simulink model "gm_sampleModel1519_4_sub"  (R2023a)
settings: Solver=VariableStepAuto  StartTime=0.0  StopTime=10.0  RelTol=1e-3
libraries: simulink x2
settings Model: Creator=user1  LastModifiedBy=user1
settings OptimizationCC: BlockReduction=off  ConditionallyExecuteInputs=off
settings DebuggingCC: InheritedTsInSrcMsg=none

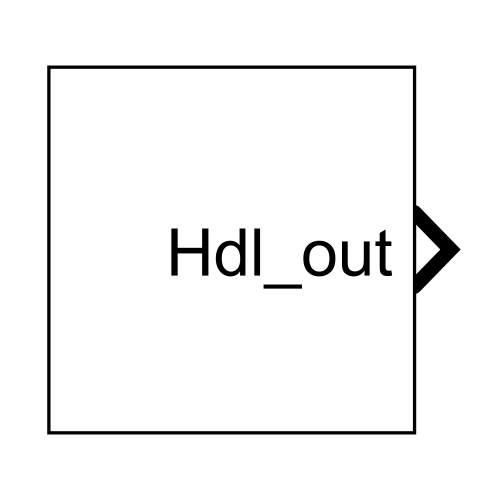
[thumbnail: Simulink's stored preview of the top-level diagram]
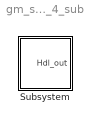
== system gm_sampleModel1519_4_sub ==
  Subsystem : Subsystem

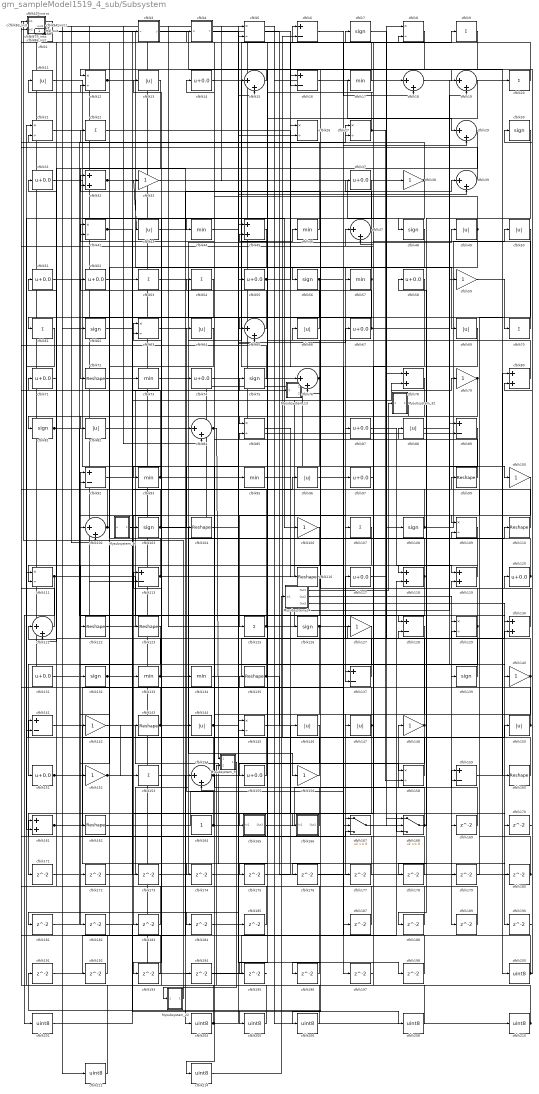
== system gm_sampleModel1519_4_sub/Subsystem ==
  Mysubsystem_13 : Subsystem
  Mysubsystem_22 : Subsystem
  Mysubsystem_32 : Subsystem
  Mysubsystem_34 : Subsystem
  Mysubsystem_36 : Subsystem
  Mysubsystem_9 : Subsystem
  cfblk1 : simulink/Logic and Bit Operations/Detect Increase  vinit=0.0  OutDataTypeStr=uint8
      settings: LibrarySourceBlock=|
      | hdlsllib/Logic and Bit
      | Operations/Detect
      | Increase
  cfblk{33,38,59,79,100,106,127,140,142,148,152,156} (12 alike) : Gain  OutDataTypeStr=uint8
  cfblk{15,18..19,29,39,47,65,76,84,102,121,154} (12 alike) : Sum  Inputs=|++  OutDataTypeStr=uint8
  cfblk{7,30,48,56,62,75,81,103,108,126,132,139} (12 alike) : Signum
  cfblk{72,99,104,110,116,122..123,135,143,160,162} (11 alike) : Reshape
  cfblk105_inst : Subsystem
  cfblk{9,20,22,53..54,61,70,107,125,153} (10 alike) : Sum  Inputs=+  OutDataTypeStr=uint8
  cfblk{5,8,12,21,26..27,42,63,85,109,111,129,145,158} (14 alike) : Product  Inputs=*/  OutDataTypeStr=uint8  RndMeth=Zero  SaturateOnIntegerOverflow=on
  cfblk{11,13,43,49..50,64,66,69,82,88,96,144,146..147,150} (15 alike) : Abs  OutDataTypeStr=uint8  SaturateOnIntegerOverflow=off
  cfblk112_inst : Subsystem
  cfblk{6,16,89,92,113,128,137,141,159} (9 alike) : Sum  Inputs=+-  OutDataTypeStr=uint8
  cfblk114_inst : Subsystem
  cfblk{14,31,37,51..52,55,58,67,71,74,87,97,117,120,131,151,155} (17 alike) : Bias  Bias=0.0  SaturateOnIntegerOverflow=off
  cfblk{32,45,78,80,118..119,130,161} (8 alike) : Sum  OutDataTypeStr=uint8
  cfblk124_inst : Subsystem
  cfblk{17,44,46,57,73,93,95,133..134} (9 alike) : MinMax  OutDataTypeStr=uint8
  cfblk149_inst : Subsystem
  cfblk157_inst : Subsystem
  cfblk164 : Constant  OutDataTypeStr=uint8  SampleTime=-1
  cfblk165 : Subsystem
  cfblk166 : Subsystem
  cfblk167 : Switch  OutDataTypeStr=uint8  SaturateOnIntegerOverflow=off  InputSameDT=off
  cfblk168 : Switch  OutDataTypeStr=uint8  SaturateOnIntegerOverflow=off  InputSameDT=off
  cfblk{169..185,187..198} (29 alike) : Delay  SampleTime=1
  cfblk{200..201,204..206,208,210,212,214} (9 alike) : DataTypeConversion  OutDataTypeStr=uint8  SaturateOnIntegerOverflow=off  RndMeth=Floor
  cfblk24_inst : Subsystem
  cfblk25_inst : Subsystem
  cfblk3 : Subsystem  mask(Compare To Zero){relop=<=, OutDataTypeStr=uint8, ZeroCross=on}
      mask prompts: relop "Simulink:masks:Operator_MP"; OutDataTypeStr "Simulink:masks:OutputDataType_MP"; ZeroCross "Simulink:masks:EnableZerocrossingDetection_MP"
      mask help: Simulink:masks:CompareToZero_MD
      mask init:
      | OutDataTypeStr = 'uint8';
      | ZeroCross = 'on';
      | blkName = 'sampleModel1519_4_sub/Subsystem/cfblk3';
      | relop = '<=';
      | setValue = 'fixdt(0, 8)';
      mask TypeOptions relop: == | ~= | < | <= | >= | >
      mask TypeOptions OutDataTypeStr: Simulink:masks:uint8 | Simulink:masks:boolean
      mask Callback ZeroCross: sl('zeroCrossEnable', gcbh);
      mask Display: disp([relop,' 0'])
  cfblk34_inst : Subsystem
  cfblk36_inst : Subsystem
  cfblk4 : Subsystem  mask(Detect Rise Positive){vinit=double(0), InputProcessing=Elements as channels (sample based), OutDataTypeStr=uint8}
      mask prompts: vinit "Simulink:masks:InitialCondition_MP"; InputProcessing "Simulink:masks:InputProcessing_MP"; OutDataTypeStr "Simulink:masks:OutputDataType_MP"
      mask help: Simulink:masks:DetectRisePositive_MD
      mask init:
      | InputProcessing = 'Elements as channels (sample based)';
      | OutDataTypeStr = 'uint8';
      | vinit = double(0);
      mask TypeOptions InputProcessing: Simulink:masks:ColumnsAsChannelsFrameBased | Simulink:masks:ElementsAsChannelsSampleBased
      mask TypeOptions OutDataTypeStr: Simulink:masks:uint8 | Simulink:masks:boolean
      mask Display: fprintf('U > 0\n&  NOT\nU/z > 0')
  cfblk41_inst : Subsystem
  cfblk77_inst : Subsystem
  cfblk83_inst : Subsystem
  cfblk86_inst : Subsystem
  cfblk94_inst : Subsystem
  Hdl_out : Outport  OutDataTypeStr=uint8  SampleTime=1
  wires:
  Mysubsystem_13/1(Out1) -> Mysubsystem_36/1(u)
  Mysubsystem_13/2(Out2) -> cfblk184/1
  Mysubsystem_22/1(Out1) -> cfblk34_inst/1(in1)
  Mysubsystem_32/1(Out1) -> cfblk191/1
  Mysubsystem_34/1(Out1) -> Mysubsystem_32/1(In1)
  Mysubsystem_34/2(Out2) -> cfblk189/1
  Mysubsystem_34/3(Out3) -> cfblk190/1
  Mysubsystem_36/1(Out1) -> cfblk183/1
  Mysubsystem_9/1(Out1) -> Mysubsystem_22/1(In1)
  cfblk1/1 -> cfblk44/1
  cfblk100/1 -> cfblk125/1
  cfblk102/1 -> cfblk25_inst/2(in2), cfblk27/1
  cfblk103/1 -> cfblk114_inst/2(in2), cfblk156/1, cfblk109/2
  cfblk104/1 -> cfblk145/1
  cfblk105_inst/1(out1) -> cfblk149_inst/2(in2)
  cfblk106/1 -> cfblk111/2
  cfblk107/1 -> cfblk165/1(In1)
  cfblk108/1 -> cfblk92/1, cfblk50/1
  cfblk109/1 -> cfblk182/1
  cfblk11/1 -> cfblk185/1
  cfblk110/1 -> cfblk24_inst/2(in2)
  cfblk111/1 -> cfblk201/1, cfblk130/1
  cfblk112_inst/1(out1) -> cfblk84/2, cfblk212/1
  cfblk113/1 -> cfblk78/2, cfblk11/1
  cfblk114_inst/1(out1) -> cfblk53/1
  cfblk116/1 -> cfblk172/1
  cfblk117/1 -> cfblk8/1
  cfblk118/1 -> cfblk71/1, cfblk12/2, cfblk153/1
  cfblk119/1 -> cfblk118/1
  cfblk12/1 -> cfblk69/1, cfblk137/2
  cfblk120/1 -> cfblk94_inst/1(in1), cfblk157_inst/2(in2)
  cfblk121/1 -> cfblk83_inst/2(in2)
  cfblk122/1 -> cfblk75/1
  cfblk123/1 -> cfblk132/1
  cfblk124_inst/1(out1) -> cfblk38/1
  cfblk125/1 -> cfblk19/2, cfblk13/1
  cfblk126/1 -> cfblk214/1, cfblk130/2
  cfblk127/1 -> cfblk151/1
  cfblk128/1 -> cfblk177/1
  cfblk129/1 -> cfblk88/1, cfblk76/2, cfblk155/1
  cfblk13/1 -> cfblk72/1
  cfblk130/1 -> cfblk32/1
  cfblk131/1 -> cfblk133/1
  cfblk132/1 -> cfblk79/1, cfblk179/1
  cfblk133/1 -> cfblk92/2, cfblk49/1
  cfblk134/1 -> cfblk78/1
  cfblk135/1 -> cfblk64/1, cfblk146/1
  cfblk137/1 -> cfblk157_inst/1(in1)
  cfblk139/1 -> cfblk58/1
  cfblk14/1 -> cfblk168/1
  cfblk140/1 -> cfblk99/1, cfblk154/2
  cfblk141/1 -> cfblk194/1
  cfblk142/1 -> cfblk180/1
  cfblk143/1 -> cfblk6/1, cfblk21/2
  cfblk144/1 -> cfblk67/1, cfblk14/1
  cfblk145/1 -> cfblk169/1
  cfblk146/1 -> cfblk181/1
  cfblk147/1 -> cfblk7/1, cfblk51/1, cfblk85/2, cfblk171/1
  cfblk148/1 -> cfblk117/1, cfblk176/1
  cfblk149_inst/1(out1) -> cfblk131/1
  cfblk15/1 -> cfblk12/1
  cfblk150/1 -> cfblk41_inst/2(in2), cfblk27/2
  cfblk151/1 -> cfblk150/1, cfblk73/1
  cfblk152/1 -> cfblk96/1, cfblk143/1
  cfblk153/1 -> cfblk46/1
  cfblk154/1 -> cfblk113/1, cfblk26/2
  cfblk155/1 -> cfblk21/1
  cfblk156/1 -> cfblk74/1
  cfblk157_inst/1(out1) -> cfblk126/1
  cfblk158/1 -> cfblk135/1
  cfblk159/1 -> cfblk80/1
  cfblk16/1 -> cfblk29/1
  cfblk160/1 -> cfblk141/1
  cfblk161/1 -> cfblk15/2, cfblk17/1
  cfblk162/1 -> cfblk97/1
  cfblk164/1 -> cfblk144/1, cfblk110/1
  cfblk165/1(Out1) -> cfblk148/1
  cfblk166/1(Out1) -> cfblk86_inst/1(in1)
  cfblk167/1 -> cfblk159/1
  cfblk168/1 -> cfblk128/2, cfblk42/1, cfblk127/1
  cfblk169/1 -> cfblk159/2
  cfblk17/1 -> cfblk36_inst/2(in2)
  cfblk170/1 -> cfblk19/1
  cfblk171/1 -> cfblk167/3
  cfblk172/1 -> cfblk65/2
  cfblk173/1 -> cfblk6/2
  cfblk174/1 -> cfblk5/2
  cfblk175/1 -> cfblk18/1
  cfblk176/1 -> cfblk29/2
  cfblk177/1 -> cfblk105_inst/1(in1)
  cfblk178/1 -> cfblk45/2
  cfblk179/1 -> cfblk119/2
  cfblk18/1 -> cfblk140/1
  cfblk180/1 -> cfblk129/2, Hdl_out/1
  cfblk181/1 -> cfblk26/1
  cfblk182/1 -> cfblk205/1
  cfblk183/1 -> cfblk77_inst/2(in2)
  cfblk184/1 -> cfblk39/2
  cfblk185/1 -> cfblk161/1
  cfblk187/1 -> cfblk36_inst/1(in1)
  cfblk188/1 -> cfblk121/1
  cfblk189/1 -> cfblk112_inst/2(in2)
  cfblk19/1 -> cfblk65/1
  cfblk190/1 -> cfblk80/2
  cfblk191/1 -> cfblk154/1
  cfblk192/1 -> cfblk124_inst/2(in2)
  cfblk193/1 -> cfblk83_inst/1(in1)
  cfblk194/1 -> cfblk118/2
  cfblk195/1 -> cfblk1/1
  cfblk196/1 -> cfblk149_inst/1(in1)
  cfblk197/1 -> cfblk47/2
  cfblk198/1 -> cfblk167/2
  cfblk20/1 -> cfblk124_inst/1(in1)
  cfblk200/1 -> cfblk30/1, cfblk120/1, cfblk102/1
  cfblk201/1 -> cfblk3/1(u)
  cfblk204/1 -> cfblk77_inst/1(in1), cfblk15/1
  cfblk205/1 -> cfblk63/1
  cfblk206/1 -> cfblk63/2
  cfblk208/1 -> Mysubsystem_9/2(In2)
  cfblk21/1 -> cfblk84/1
  cfblk210/1 -> cfblk86_inst/2(in2), cfblk47/1, cfblk111/1
  cfblk212/1 -> cfblk34_inst/2(in2)
  cfblk214/1 -> Mysubsystem_34/1(In1)
  cfblk22/1 -> cfblk87/1
  cfblk24_inst/1(out1) -> cfblk162/1
  cfblk25_inst/1(out1) -> cfblk62/1, cfblk113/2
  cfblk26/1 -> cfblk56/1
  cfblk27/1 -> cfblk25_inst/1(in1), cfblk158/2
  cfblk29/1 -> cfblk121/2
  cfblk3/1(y) -> cfblk200/1
  cfblk30/1 -> cfblk188/1
  cfblk31/1 -> cfblk106/1
  cfblk32/1 -> cfblk43/1, cfblk95/1
  cfblk33/1 -> cfblk108/1
  cfblk34_inst/1(out1) -> cfblk210/1
  cfblk36_inst/1(out1) -> cfblk76/1, cfblk102/2
  cfblk37/1 -> cfblk103/1
  cfblk38/1 -> cfblk48/1, cfblk141/2, cfblk22/1
  cfblk39/1 -> cfblk24_inst/1(in1)
  cfblk4/1(Y) -> cfblk158/1
  cfblk41_inst/1(out1) -> cfblk123/1
  cfblk42/1 -> cfblk174/1, cfblk173/1
  cfblk43/1 -> cfblk39/1
  cfblk44/1 -> cfblk139/1
  cfblk45/1 -> cfblk152/1
  cfblk46/1 -> cfblk105_inst/2(in2)
  cfblk47/1 -> cfblk37/1, cfblk57/1
  cfblk48/1 -> cfblk85/1
  cfblk49/1 -> cfblk206/1, cfblk4/1(U)
  cfblk5/1 -> cfblk16/2
  cfblk50/1 -> cfblk109/1
  cfblk51/1 -> cfblk89/1
  cfblk52/1 -> cfblk129/1
  cfblk53/1 -> cfblk160/1
  cfblk54/1 -> cfblk82/1
  cfblk55/1 -> cfblk197/1, cfblk195/1, cfblk9/1
  cfblk56/1 -> cfblk8/2, cfblk61/1, cfblk93/1
  cfblk57/1 -> cfblk114_inst/1(in1), cfblk193/1
  cfblk58/1 -> cfblk167/1
  cfblk59/1 -> cfblk70/1
  cfblk6/1 -> cfblk18/2
  cfblk61/1 -> cfblk161/2
  cfblk62/1 -> cfblk33/1
  cfblk63/1 -> cfblk204/1
  cfblk64/1 -> cfblk142/1
  cfblk65/1 -> cfblk45/1
  cfblk66/1 -> cfblk52/1
  cfblk67/1 -> cfblk59/1, cfblk42/2
  cfblk69/1 -> cfblk137/1
  cfblk7/1 -> cfblk168/2
  cfblk70/1 -> cfblk16/1
  cfblk71/1 -> cfblk31/1
  cfblk72/1 -> cfblk166/1(In1)
  cfblk73/1 -> cfblk208/1
  cfblk74/1 -> cfblk55/1
  cfblk75/1 -> cfblk41_inst/1(in1)
  cfblk76/1 -> cfblk104/1, cfblk5/1
  cfblk77_inst/1(out1) -> cfblk112_inst/1(in1)
  cfblk78/1 -> cfblk122/1
  cfblk79/1 -> cfblk81/1, cfblk178/1
  cfblk8/1 -> cfblk175/1
  cfblk80/1 -> cfblk66/1
  cfblk81/1 -> cfblk128/1, cfblk107/1
  cfblk82/1 -> cfblk134/1
  cfblk83_inst/1(out1) -> cfblk20/1
  cfblk84/1 -> Mysubsystem_9/1(In1), cfblk54/1
  cfblk85/1 -> cfblk116/1
  cfblk86_inst/1(out1) -> cfblk89/2
  cfblk87/1 -> cfblk119/1
  cfblk88/1 -> cfblk100/1
  cfblk89/1 -> cfblk145/2
  cfblk9/1 -> cfblk196/1
  cfblk92/1 -> Mysubsystem_13/1(In1)
  cfblk93/1 -> cfblk94_inst/2(in2), cfblk168/3, cfblk198/1
  cfblk94_inst/1(out1) -> cfblk192/1
  cfblk95/1 -> cfblk187/1
  cfblk96/1 -> cfblk170/1
  cfblk97/1 -> cfblk147/1
  cfblk99/1 -> cfblk32/2

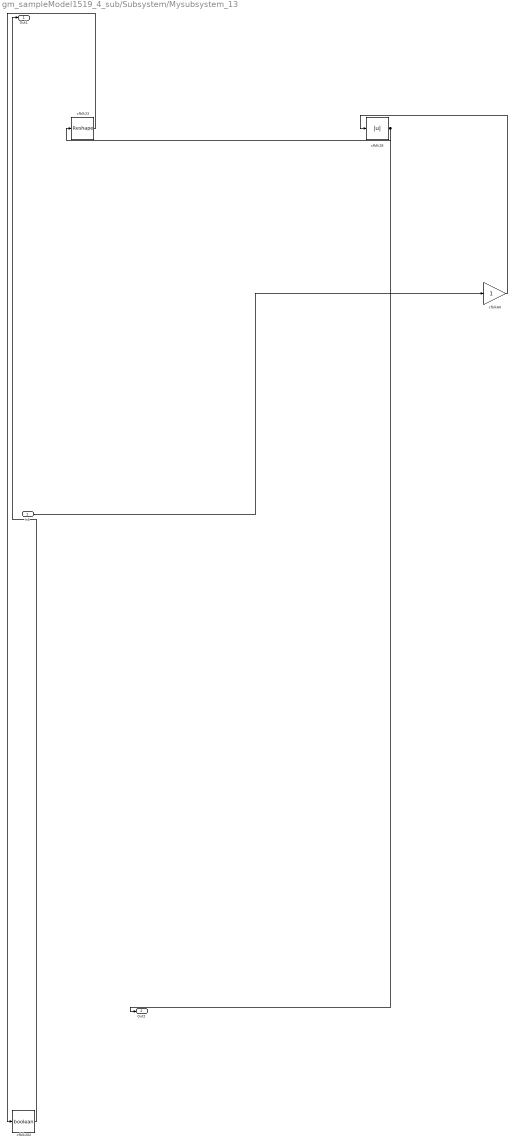
== system gm_sampleModel1519_4_sub/Subsystem/Mysubsystem_13 ==
  In1 : Inport  OutDataTypeStr=uint8  PortDimensions=1  SampleTime=1
  cfblk202 : DataTypeConversion  OutDataTypeStr=boolean  SaturateOnIntegerOverflow=off  RndMeth=Floor
  cfblk23 : Reshape
  cfblk28 : Abs  SaturateOnIntegerOverflow=off
  cfblk60 : Gain
  Out1 : Outport  SampleTime=1
  Out2 : Outport  Port=2  SampleTime=1
  wires:
  In1/1 -> cfblk60/1
  cfblk202/1 -> Out1/1
  cfblk23/1 -> cfblk202/1
  cfblk28/1 -> cfblk23/1, Out2/1
  cfblk60/1 -> cfblk28/1

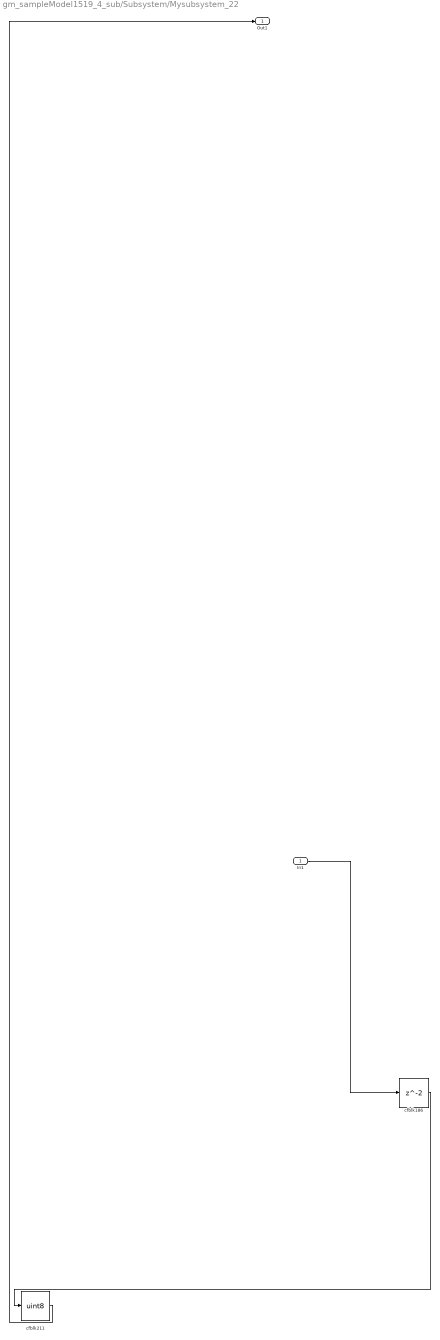
== system gm_sampleModel1519_4_sub/Subsystem/Mysubsystem_22 ==
  In1 : Inport  OutDataTypeStr=uint8  PortDimensions=1  SampleTime=1
  cfblk186 : Delay  SampleTime=1
  cfblk211 : DataTypeConversion  OutDataTypeStr=uint8  SaturateOnIntegerOverflow=off  RndMeth=Floor
  Out1 : Outport  SampleTime=1
  wires:
  In1/1 -> cfblk186/1
  cfblk186/1 -> cfblk211/1
  cfblk211/1 -> Out1/1

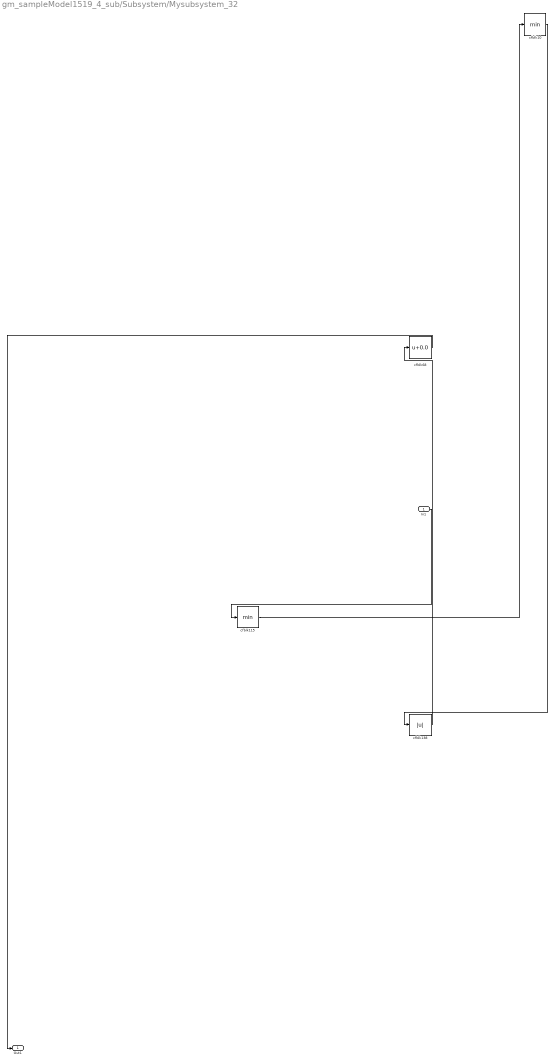
== system gm_sampleModel1519_4_sub/Subsystem/Mysubsystem_32 ==
  In1 : Inport  OutDataTypeStr=uint8  PortDimensions=1  SampleTime=1
  cfblk10 : MinMax
  cfblk115 : MinMax
  cfblk138 : Abs  SaturateOnIntegerOverflow=off
  cfblk68 : Bias  Bias=0.0  SaturateOnIntegerOverflow=off
  Out1 : Outport  SampleTime=1
  wires:
  In1/1 -> cfblk115/1
  cfblk10/1 -> cfblk138/1
  cfblk115/1 -> cfblk10/1
  cfblk138/1 -> cfblk68/1
  cfblk68/1 -> Out1/1

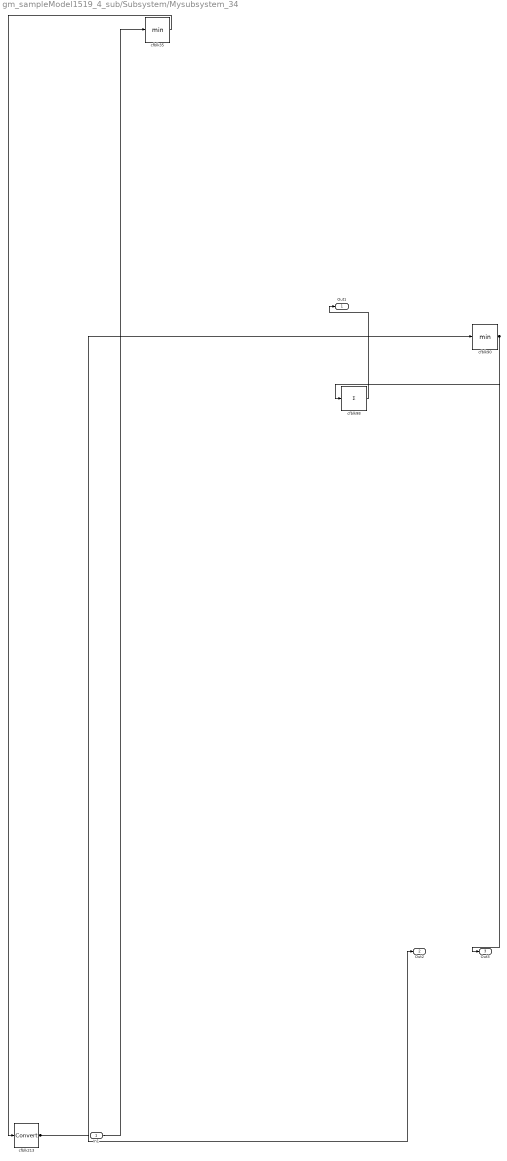
== system gm_sampleModel1519_4_sub/Subsystem/Mysubsystem_34 ==
  In1 : Inport  OutDataTypeStr=uint8  PortDimensions=1  SampleTime=1
  cfblk213 : DataTypeConversion  SaturateOnIntegerOverflow=off  RndMeth=Floor
  cfblk35 : MinMax
  cfblk90 : MinMax
  cfblk98 : Sum  Inputs=+
  Out1 : Outport  SampleTime=1
  Out2 : Outport  Port=2  SampleTime=1
  Out3 : Outport  Port=3  SampleTime=1
  wires:
  In1/1 -> cfblk35/1
  cfblk213/1 -> Out2/1, cfblk90/1
  cfblk35/1 -> cfblk213/1
  cfblk90/1 -> Out3/1, cfblk98/1
  cfblk98/1 -> Out1/1

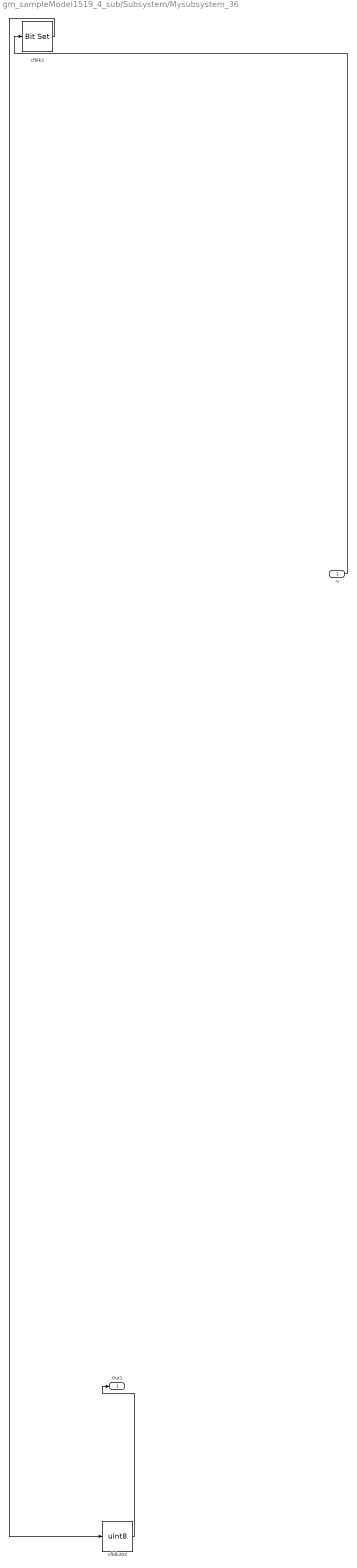
== system gm_sampleModel1519_4_sub/Subsystem/Mysubsystem_36 ==
  u : Inport  OutDataTypeStr=boolean  PortDimensions=1  SampleTime=1
  cfblk2 : simulink/Logic and Bit Operations/Bit Set  iBit=0
      settings: LibrarySourceBlock=|
      | hdlsllib/Logic and Bit
      | Operations/Bit Set
  cfblk203 : DataTypeConversion  OutDataTypeStr=uint8  SaturateOnIntegerOverflow=off  RndMeth=Floor
  Out1 : Outport  SampleTime=1
  wires:
  u/1 -> cfblk2/1
  cfblk2/1 -> cfblk203/1
  cfblk203/1 -> Out1/1

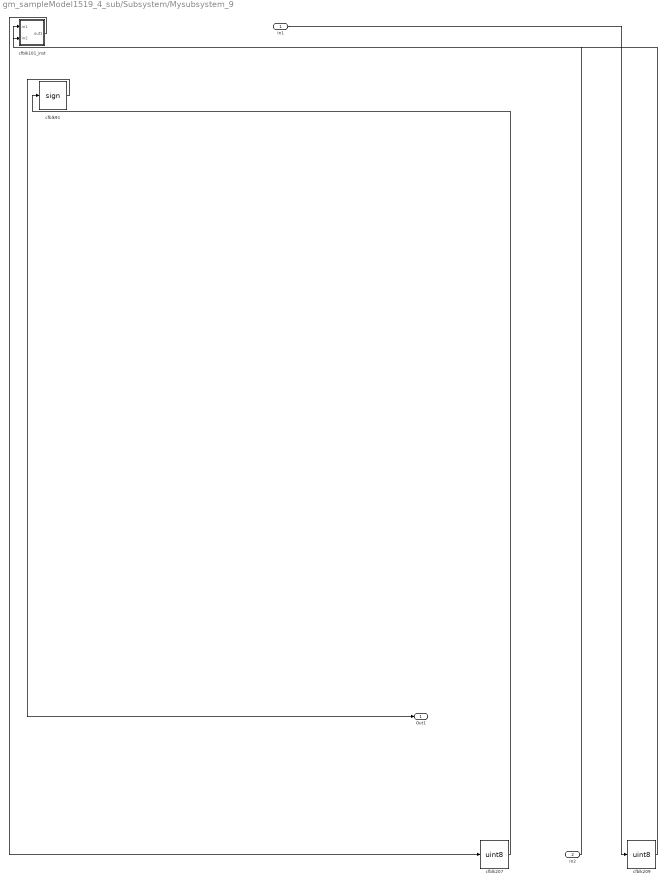
== system gm_sampleModel1519_4_sub/Subsystem/Mysubsystem_9 ==
  In1 : Inport  OutDataTypeStr=uint8  PortDimensions=1  SampleTime=1
  In2 : Inport  Port=2  OutDataTypeStr=uint8  PortDimensions=1  SampleTime=1
  cfblk101_inst : Subsystem
  cfblk207 : DataTypeConversion  OutDataTypeStr=uint8  SaturateOnIntegerOverflow=off  RndMeth=Floor
  cfblk209 : DataTypeConversion  OutDataTypeStr=uint8  SaturateOnIntegerOverflow=off  RndMeth=Floor
  cfblk91 : Signum
  Out1 : Outport  SampleTime=1
  wires:
  In1/1 -> cfblk209/1
  In2/1 -> cfblk101_inst/1(in1)
  cfblk101_inst/1(out1) -> cfblk207/1
  cfblk207/1 -> cfblk91/1
  cfblk209/1 -> cfblk101_inst/2(in2)
  cfblk91/1 -> Out1/1

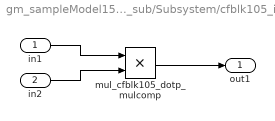
== system gm_sampleModel1519_4_sub/Subsystem/cfblk105_inst ==
  in1 : Inport  OutDataTypeStr=uint8  SampleTime=1
  in2 : Inport  Port=2  OutDataTypeStr=uint8  SampleTime=1
  mul_cfblk105_dotp_mulcomp : Product  Inputs=**  OutDataTypeStr=uint8  SampleTime=1
  out1 : Outport  OutDataTypeStr=uint8  SampleTime=1
  wires:
  in1/1 -> mul_cfblk105_dotp_mulcomp/1
  in2/1 -> mul_cfblk105_dotp_mulcomp/2
  mul_cfblk105_dotp_mulcomp/1 -> out1/1

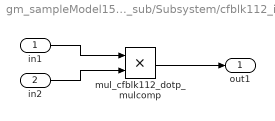
== system gm_sampleModel1519_4_sub/Subsystem/cfblk112_inst ==
  in1 : Inport  OutDataTypeStr=uint8  SampleTime=1
  in2 : Inport  Port=2  OutDataTypeStr=uint8  SampleTime=1
  mul_cfblk112_dotp_mulcomp : Product  Inputs=**  OutDataTypeStr=uint8  SampleTime=1
  out1 : Outport  OutDataTypeStr=uint8  SampleTime=1
  wires:
  in1/1 -> mul_cfblk112_dotp_mulcomp/1
  in2/1 -> mul_cfblk112_dotp_mulcomp/2
  mul_cfblk112_dotp_mulcomp/1 -> out1/1

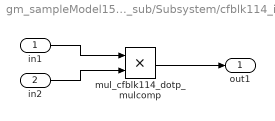
== system gm_sampleModel1519_4_sub/Subsystem/cfblk114_inst ==
  in1 : Inport  OutDataTypeStr=uint8  SampleTime=1
  in2 : Inport  Port=2  OutDataTypeStr=uint8  SampleTime=1
  mul_cfblk114_dotp_mulcomp : Product  Inputs=**  OutDataTypeStr=uint8  SampleTime=1
  out1 : Outport  OutDataTypeStr=uint8  SampleTime=1
  wires:
  in1/1 -> mul_cfblk114_dotp_mulcomp/1
  in2/1 -> mul_cfblk114_dotp_mulcomp/2
  mul_cfblk114_dotp_mulcomp/1 -> out1/1

== system gm_sampleModel1519_4_sub/Subsystem/cfblk124_inst ==
  in1 : Inport  OutDataTypeStr=uint8  SampleTime=1
  in2 : Inport  Port=2  OutDataTypeStr=uint8  SampleTime=1
  mul_cfblk124_dotp_mulcomp : Product  Inputs=**  OutDataTypeStr=uint8  SampleTime=1
  out1 : Outport  OutDataTypeStr=uint8  SampleTime=1
  wires:
  in1/1 -> mul_cfblk124_dotp_mulcomp/1
  in2/1 -> mul_cfblk124_dotp_mulcomp/2
  mul_cfblk124_dotp_mulcomp/1 -> out1/1

== system gm_sampleModel1519_4_sub/Subsystem/cfblk149_inst ==
  in1 : Inport  OutDataTypeStr=uint8  SampleTime=1
  in2 : Inport  Port=2  OutDataTypeStr=uint8  SampleTime=1
  mul_cfblk149_dotp_mulcomp : Product  Inputs=**  OutDataTypeStr=uint8  SampleTime=1
  out1 : Outport  OutDataTypeStr=uint8  SampleTime=1
  wires:
  in1/1 -> mul_cfblk149_dotp_mulcomp/1
  in2/1 -> mul_cfblk149_dotp_mulcomp/2
  mul_cfblk149_dotp_mulcomp/1 -> out1/1

== system gm_sampleModel1519_4_sub/Subsystem/cfblk157_inst ==
  in1 : Inport  OutDataTypeStr=uint8  SampleTime=1
  in2 : Inport  Port=2  OutDataTypeStr=uint8  SampleTime=1
  mul_cfblk157_dotp_mulcomp : Product  Inputs=**  OutDataTypeStr=uint8  SampleTime=1
  out1 : Outport  OutDataTypeStr=uint8  SampleTime=1
  wires:
  in1/1 -> mul_cfblk157_dotp_mulcomp/1
  in2/1 -> mul_cfblk157_dotp_mulcomp/2
  mul_cfblk157_dotp_mulcomp/1 -> out1/1

== system gm_sampleModel1519_4_sub/Subsystem/cfblk165 ==
  In1 : Inport  OutDataTypeStr=uint8  PortDimensions=1  SampleTime=1
  Out1 : Outport  SampleTime=1
  wires:
  In1/1 -> Out1/1

== system gm_sampleModel1519_4_sub/Subsystem/cfblk166 ==
  In1 : Inport  OutDataTypeStr=uint8  PortDimensions=1  SampleTime=1
  Out1 : Outport  SampleTime=1
  wires:
  In1/1 -> Out1/1

== system gm_sampleModel1519_4_sub/Subsystem/cfblk24_inst ==
  in1 : Inport  OutDataTypeStr=uint8  SampleTime=1
  in2 : Inport  Port=2  OutDataTypeStr=uint8  SampleTime=1
  mul_cfblk24_dotp_mulcomp : Product  Inputs=**  OutDataTypeStr=uint8  SampleTime=1
  out1 : Outport  OutDataTypeStr=uint8  SampleTime=1
  wires:
  in1/1 -> mul_cfblk24_dotp_mulcomp/1
  in2/1 -> mul_cfblk24_dotp_mulcomp/2
  mul_cfblk24_dotp_mulcomp/1 -> out1/1

== system gm_sampleModel1519_4_sub/Subsystem/cfblk25_inst ==
  in1 : Inport  OutDataTypeStr=uint8  SampleTime=1
  in2 : Inport  Port=2  OutDataTypeStr=uint8  SampleTime=1
  mul_cfblk25_dotp_mulcomp : Product  Inputs=**  OutDataTypeStr=uint8  SampleTime=1
  out1 : Outport  OutDataTypeStr=uint8  SampleTime=1
  wires:
  in1/1 -> mul_cfblk25_dotp_mulcomp/1
  in2/1 -> mul_cfblk25_dotp_mulcomp/2
  mul_cfblk25_dotp_mulcomp/1 -> out1/1

== system gm_sampleModel1519_4_sub/Subsystem/cfblk3 ==
  u : Inport  OutDataTypeStr=uint8  SampleTime=1
  Compare : RelationalOperator  Operator=<=  OutDataTypeStr=fixdt(0, 8)
  Constant : Constant  DisableCoverage=on  Value=0  OutDataTypeStr=Inherit: Inherit via back propagation  SampleTime=-1  PreserveConstantTs=on
  y : Outport  SampleTime=1
  wires:
  u/1 -> Compare/1
  Compare/1 -> y/1
  Constant/1 -> Compare/2

== system gm_sampleModel1519_4_sub/Subsystem/cfblk34_inst ==
  in1 : Inport  OutDataTypeStr=uint8  SampleTime=1
  in2 : Inport  Port=2  OutDataTypeStr=uint8  SampleTime=1
  mul_cfblk34_dotp_mulcomp : Product  Inputs=**  OutDataTypeStr=uint8  SampleTime=1
  out1 : Outport  OutDataTypeStr=uint8  SampleTime=1
  wires:
  in1/1 -> mul_cfblk34_dotp_mulcomp/1
  in2/1 -> mul_cfblk34_dotp_mulcomp/2
  mul_cfblk34_dotp_mulcomp/1 -> out1/1

== system gm_sampleModel1519_4_sub/Subsystem/cfblk36_inst ==
  in1 : Inport  OutDataTypeStr=uint8  SampleTime=1
  in2 : Inport  Port=2  OutDataTypeStr=uint8  SampleTime=1
  mul_cfblk36_dotp_mulcomp : Product  Inputs=**  OutDataTypeStr=uint8  SampleTime=1
  out1 : Outport  OutDataTypeStr=uint8  SampleTime=1
  wires:
  in1/1 -> mul_cfblk36_dotp_mulcomp/1
  in2/1 -> mul_cfblk36_dotp_mulcomp/2
  mul_cfblk36_dotp_mulcomp/1 -> out1/1

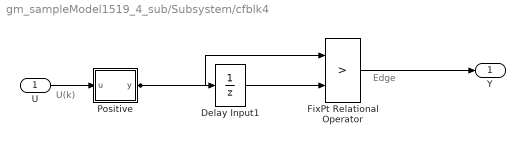
== system gm_sampleModel1519_4_sub/Subsystem/cfblk4 ==
  note: U(k)
  note: Edge
  U : Inport  OutDataTypeStr=uint8  SampleTime=1
  Delay Input1 : UnitDelay  Description=Store in Global RAM  DisableCoverage=on  InitialCondition=vinit  SampleTime=-1  HasFrameUpgradeWarning=on
  FixPt Relational Operator : RelationalOperator  Operator=>  OutDataTypeStr=fixdt(0, 8)  ZeroCross=off  InputSameDT=off
  Positive : Subsystem  mask(Compare To Zero){relop=>, OutDataTypeStr=boolean, ZeroCross=off}
      mask prompts: relop "Simulink:masks:Operator_MP"; OutDataTypeStr "Simulink:masks:OutputDataType_MP"; ZeroCross "Simulink:masks:EnableZerocrossingDetection_MP"
      mask help: Simulink:masks:CompareToZero_MD
      mask init:
      | OutDataTypeStr = 'boolean';
      | ZeroCross = 'off';
      | blkName = 'sampleModel1519_4_sub/Subsystem/cfblk4/Positive';
      | relop = '>';
      | setValue = 'boolean';
      mask TypeOptions relop: == | ~= | < | <= | >= | >
      mask TypeOptions OutDataTypeStr: Simulink:masks:uint8 | Simulink:masks:boolean
      mask Callback ZeroCross: sl('zeroCrossEnable', gcbh);
      mask Display: disp([relop,' 0'])
  Y : Outport  SampleTime=1
  wires:
  U/1 -> Positive/1(u)
  Delay Input1/1 -> FixPt Relational Operator/2
  FixPt Relational Operator/1 -> Y/1
  Positive/1(y) -> FixPt Relational Operator/1, Delay Input1/1

== system gm_sampleModel1519_4_sub/Subsystem/cfblk41_inst ==
  in1 : Inport  OutDataTypeStr=uint8  SampleTime=1
  in2 : Inport  Port=2  OutDataTypeStr=uint8  SampleTime=1
  mul_cfblk41_dotp_mulcomp : Product  Inputs=**  OutDataTypeStr=uint8  SampleTime=1
  out1 : Outport  OutDataTypeStr=uint8  SampleTime=1
  wires:
  in1/1 -> mul_cfblk41_dotp_mulcomp/1
  in2/1 -> mul_cfblk41_dotp_mulcomp/2
  mul_cfblk41_dotp_mulcomp/1 -> out1/1

== system gm_sampleModel1519_4_sub/Subsystem/cfblk77_inst ==
  in1 : Inport  OutDataTypeStr=uint8  SampleTime=1
  in2 : Inport  Port=2  OutDataTypeStr=uint8  SampleTime=1
  mul_cfblk77_dotp_mulcomp : Product  Inputs=**  OutDataTypeStr=uint8  SampleTime=1
  out1 : Outport  OutDataTypeStr=uint8  SampleTime=1
  wires:
  in1/1 -> mul_cfblk77_dotp_mulcomp/1
  in2/1 -> mul_cfblk77_dotp_mulcomp/2
  mul_cfblk77_dotp_mulcomp/1 -> out1/1

== system gm_sampleModel1519_4_sub/Subsystem/cfblk83_inst ==
  in1 : Inport  OutDataTypeStr=uint8  SampleTime=1
  in2 : Inport  Port=2  OutDataTypeStr=uint8  SampleTime=1
  mul_cfblk83_dotp_mulcomp : Product  Inputs=**  OutDataTypeStr=uint8  SampleTime=1
  out1 : Outport  OutDataTypeStr=uint8  SampleTime=1
  wires:
  in1/1 -> mul_cfblk83_dotp_mulcomp/1
  in2/1 -> mul_cfblk83_dotp_mulcomp/2
  mul_cfblk83_dotp_mulcomp/1 -> out1/1

== system gm_sampleModel1519_4_sub/Subsystem/cfblk86_inst ==
  in1 : Inport  OutDataTypeStr=uint8  SampleTime=1
  in2 : Inport  Port=2  OutDataTypeStr=uint8  SampleTime=1
  mul_cfblk86_dotp_mulcomp : Product  Inputs=**  OutDataTypeStr=uint8  SampleTime=1
  out1 : Outport  OutDataTypeStr=uint8  SampleTime=1
  wires:
  in1/1 -> mul_cfblk86_dotp_mulcomp/1
  in2/1 -> mul_cfblk86_dotp_mulcomp/2
  mul_cfblk86_dotp_mulcomp/1 -> out1/1

== system gm_sampleModel1519_4_sub/Subsystem/cfblk94_inst ==
  in1 : Inport  OutDataTypeStr=uint8  SampleTime=1
  in2 : Inport  Port=2  OutDataTypeStr=uint8  SampleTime=1
  mul_cfblk94_dotp_mulcomp : Product  Inputs=**  OutDataTypeStr=uint8  SampleTime=1
  out1 : Outport  OutDataTypeStr=uint8  SampleTime=1
  wires:
  in1/1 -> mul_cfblk94_dotp_mulcomp/1
  in2/1 -> mul_cfblk94_dotp_mulcomp/2
  mul_cfblk94_dotp_mulcomp/1 -> out1/1

== system gm_sampleModel1519_4_sub/Subsystem/Mysubsystem_9/cfblk101_inst ==
  in1 : Inport  OutDataTypeStr=uint8  SampleTime=1
  in2 : Inport  Port=2  OutDataTypeStr=uint8  SampleTime=1
  mul_cfblk101_dotp_mulcomp : Product  Inputs=**  OutDataTypeStr=uint16  SampleTime=1
  out1 : Outport  OutDataTypeStr=uint16  SampleTime=1
  wires:
  in1/1 -> mul_cfblk101_dotp_mulcomp/1
  in2/1 -> mul_cfblk101_dotp_mulcomp/2
  mul_cfblk101_dotp_mulcomp/1 -> out1/1

== system gm_sampleModel1519_4_sub/Subsystem/cfblk4/Positive ==
  u : Inport  OutDataTypeStr=uint8  SampleTime=1
  Compare : RelationalOperator  Operator=>  OutDataTypeStr=boolean  ZeroCross=off
  Constant : Constant  DisableCoverage=on  Value=0  OutDataTypeStr=Inherit: Inherit via back propagation  SampleTime=-1  PreserveConstantTs=on
  y : Outport  SampleTime=1
  wires:
  u/1 -> Compare/1
  Compare/1 -> y/1
  Constant/1 -> Compare/2
